simulink model "PID_AccuratePlant"  (R2021a)
settings: Solver=ode45  StartTime=0.0  StopTime=22  RelTol=1e-3
undefined symbols (not defined in the file): drv, gbox, kd_best, ki_best, kp_best, mld, mot, rads2rpm, sens, simp_model
libraries: spsStairGeneratorLib x1
settings Model: Creator=gioel  LastModifiedBy=gioel
settings SolverCC: AlgebraicLoopSolver=TrustRegion
settings DebuggingCC: SFMachineParentedDataDiag=warning

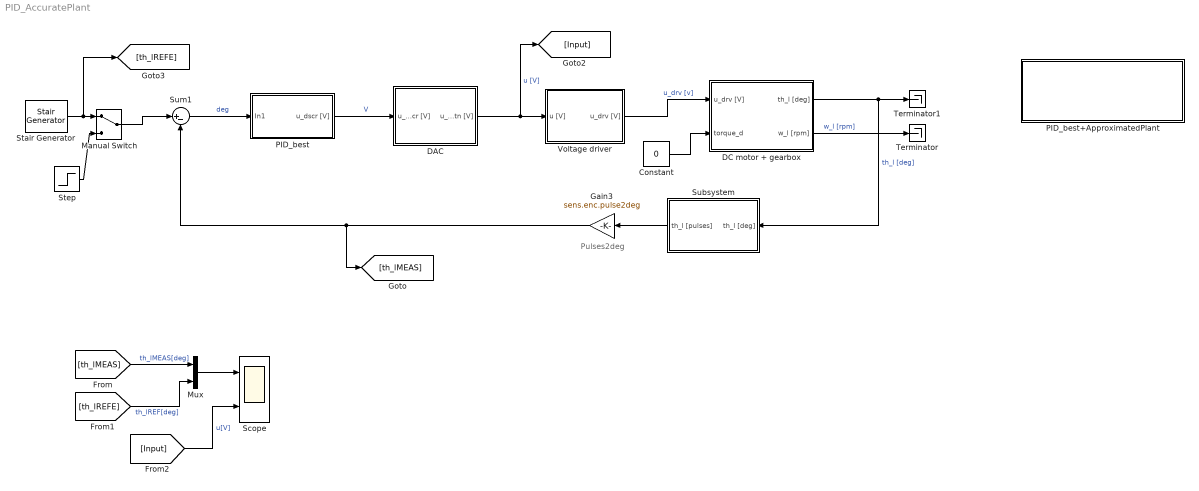
== system PID_AccuratePlant ==
  note: Pulses2deg
  Constant : Constant  Value=0
  DAC : Subsystem
  DC motor + gearbox : Subsystem
  Gain3 : Gain  Gain=sens.enc.pulse2deg
  Manual Switch : ManualSwitch
  Mux : Mux  Inputs=2
  PID_best : Subsystem
  PID_best+ApproximatedPlant : Subsystem
  Scope : Scope  NumInputPorts=2
  Stair Generator : spsStairGeneratorLib/Stair Generator  t=[0,2, 4, 6,8,10,12,14,16,18,20]  e=[10,0,30,0,50,0,90,0,180,0,360]  Ts=0
  Step : Step  Time=0  After=10  SampleTime=0
  Subsystem : Subsystem
  Sum1 : Sum  Inputs=|+-
  Terminator : Terminator
  Terminator1 : Terminator
  Voltage driver : Subsystem
  wires:
  Voltage driver/1(u_drv [V]) -> DC motor + gearbox/1(u_drv [V])  "u_drv [v]"
  DC motor + gearbox/1(th_l [deg]) -> Terminator1/1, Subsystem/1(th_l [deg])  "th_l [deg]"
  DC motor + gearbox/2(w_l [rpm]) -> Terminator/1  "w_l [rpm]"
  DAC/1(u_cntn [V]) -> [Input], Voltage driver/1(u [V])  "u [V]"
  Subsystem/1(th_l [pulses]) -> Gain3/1
  Stair Generator/1 -> [th_lREFE], Manual Switch/1
  Sum1/1 -> PID_best/1(In1)  "deg"
  Gain3/1 -> Sum1/2, [th_lMEAS]
  [th_lMEAS] -> Mux/1  "th_lMEAS[deg]"
  [th_lREFE] -> Mux/2  "th_lREF[deg]"
  [Input] -> Scope/2  "u[V]"
  Mux/1 -> Scope/1
  Step/1 -> Manual Switch/2
  Manual Switch/1 -> Sum1/1
  PID_best/1(u_dscr [V]) -> DAC/1(u_dscr [V])  "V"
  Constant/1 -> DC motor + gearbox/2(torque_d)

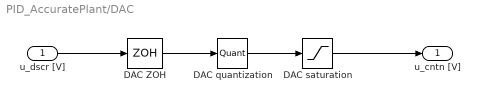
== system PID_AccuratePlant/DAC ==
  u_dscr [V] : Inport
  DAC ZOH : ZeroOrderHold  SampleTime=sens.enc.T_s
  DAC quantization : Quantizer  QuantizationInterval=daq.dac.q
  DAC saturation : Saturate  UpperLimit=10  LowerLimit=-10
  u_cntn [V] : Outport
  wires:
  DAC quantization/1 -> DAC saturation/1
  DAC ZOH/1 -> DAC quantization/1
  DAC saturation/1 -> u_cntn [V]/1
  u_dscr [V]/1 -> DAC ZOH/1

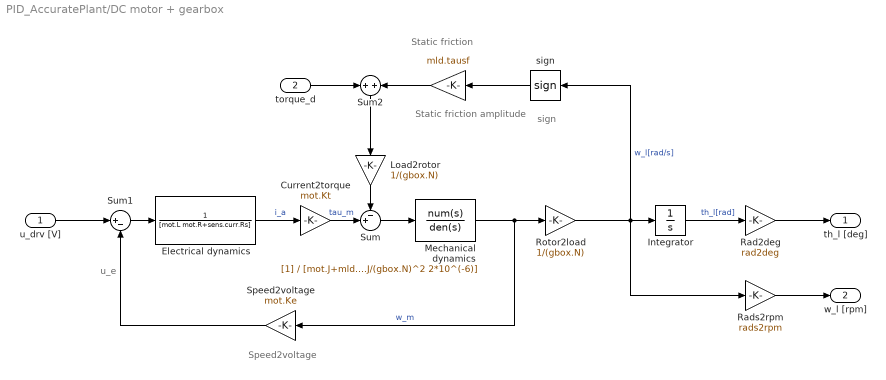
== system PID_AccuratePlant/DC motor + gearbox ==
  note: u_e
  note: Speed2voltage
  note: Static friction
  note: sign
  note: Static friction
      |  amplitude
  u_drv [V] : Inport
  torque_d : Inport  Port=2
  " " : Gain  Gain=mld.tausf
  Current2torque : Gain  Gain=mot.Kt
  Electrical dynamics : TransferFcn  Denominator=[mot.L mot.R+sens.curr.Rs]
  Integrator : Integrator
  Load2rotor : Gain  Gain=1/(gbox.N)
  Mechanical dynamics : TransferFcn  Denominator=[mot.J+mld.J/(gbox.N)^2 2*10^(-6)]
  Rad2deg : Gain  Gain=rad2deg
  Rads2rpm : Gain  Gain=rads2rpm
  Rotor2load : Gain  Gain=1/(gbox.N)
  Speed2voltage : Gain  Gain=mot.Ke
  Sum : Sum  Inputs=-+|
  Sum1 : Sum  Inputs=|+-
  Sum2 : Sum  Inputs=+|+
  sign : Signum  ZeroCross=off
  th_l [deg] : Outport
  w_l [rpm] : Outport  Port=2
  wires:
  u_drv [V]/1 -> Sum1/1
  Rads2rpm/1 -> w_l [rpm]/1
  Electrical dynamics/1 -> Current2torque/1  "i_a"
  Current2torque/1 -> Sum/2  "tau_m"
  Rad2deg/1 -> th_l [deg]/1
  sign/1 -> " "/1
  Sum1/1 -> Electrical dynamics/1
  Integrator/1 -> Rad2deg/1  "th_l[rad]"
  Sum/1 -> Mechanical dynamics/1
  Load2rotor/1 -> Sum/1
  Speed2voltage/1 -> Sum1/2
  Rotor2load/1 -> Rads2rpm/1, sign/1, Integrator/1  "w_l[rad/s]"
  Mechanical dynamics/1 -> Speed2voltage/1, Rotor2load/1  "w_m"
  " "/1 -> Sum2/2
  Sum2/1 -> Load2rotor/1
  torque_d/1 -> Sum2/1

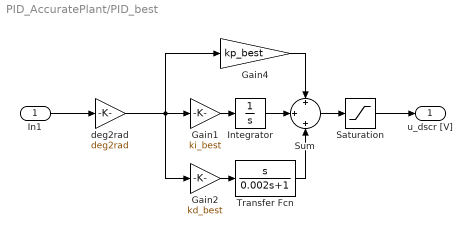
== system PID_AccuratePlant/PID_best ==
  In1 : Inport
  Gain1 : Gain  Gain=ki_best
  Gain2 : Gain  Gain=kd_best
  Gain4 : Gain  Gain=kp_best
  Integrator : Integrator
  Saturation : Saturate  UpperLimit=10  LowerLimit=-10
  Sum : Sum  Inputs=+|+|+
  Transfer Fcn : TransferFcn  Numerator=[1 0]  Denominator=[0.002 1]
  deg2rad : Gain  Gain=deg2rad
  u_dscr [V] : Outport
  wires:
  Transfer Fcn/1 -> Sum/3
  deg2rad/1 -> Gain1/1, Gain4/1, Gain2/1
  In1/1 -> deg2rad/1
  Gain2/1 -> Transfer Fcn/1
  Sum/1 -> Saturation/1
  Saturation/1 -> u_dscr [V]/1
  Integrator/1 -> Sum/2
  Gain1/1 -> Integrator/1
  Gain4/1 -> Sum/1

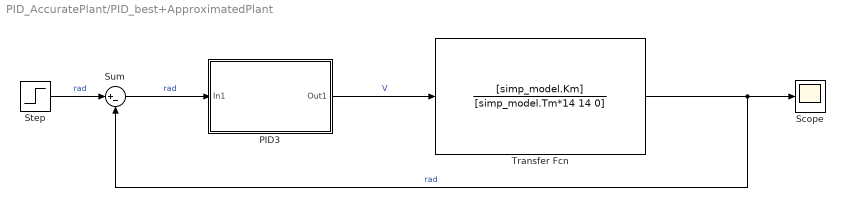
== system PID_AccuratePlant/PID_best+ApproximatedPlant ==
  PID3 : Subsystem
  Scope : Scope
  Step : Step  Time=0  SampleTime=0
  Sum : Sum  Inputs=|+-
  Transfer Fcn : TransferFcn  Numerator=[simp_model.Km]  Denominator=[simp_model.Tm*14 14 0]
  wires:
  PID3/1(Out1) -> Transfer Fcn/1  "V"
  Sum/1 -> PID3/1(In1)  "rad"
  Step/1 -> Sum/1  "rad"
  Transfer Fcn/1 -> Scope/1, Sum/2  "rad"

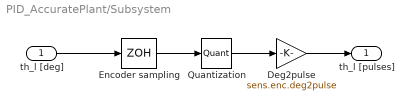
== system PID_AccuratePlant/Subsystem ==
  th_l [deg] : Inport
  Deg2pulse : Gain  Gain=sens.enc.deg2pulse
  Encoder sampling : ZeroOrderHold  SampleTime=0.001
  Quantization : Quantizer  QuantizationInterval=sens.enc.q
  th_l [pulses] : Outport
  wires:
  Encoder sampling/1 -> Quantization/1
  Quantization/1 -> Deg2pulse/1
  th_l [deg]/1 -> Encoder sampling/1
  Deg2pulse/1 -> th_l [pulses]/1

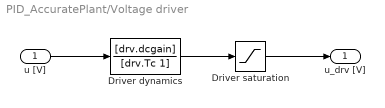
== system PID_AccuratePlant/Voltage driver ==
  u [V] : Inport
  Driver dynamics : TransferFcn  Numerator=[drv.dcgain]  Denominator=[drv.Tc 1]
  Driver saturation : Saturate  UpperLimit=12  LowerLimit=-12
  u_drv [V] : Outport
  wires:
  Driver saturation/1 -> u_drv [V]/1
  Driver dynamics/1 -> Driver saturation/1
  u [V]/1 -> Driver dynamics/1

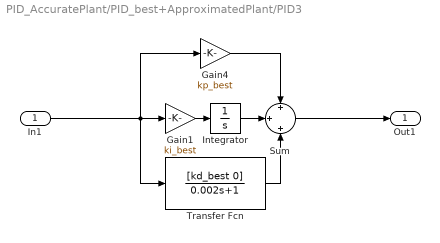
== system PID_AccuratePlant/PID_best+ApproximatedPlant/PID3 ==
  In1 : Inport
  Gain1 : Gain  Gain=ki_best
  Gain4 : Gain  Gain=kp_best
  Integrator : Integrator
  Sum : Sum  Inputs=+|+|+
  Transfer Fcn : TransferFcn  Numerator=[kd_best 0]  Denominator=[0.002 1]
  Out1 : Outport
  wires:
  Gain4/1 -> Sum/1
  Transfer Fcn/1 -> Sum/3
  In1/1 -> Gain1/1, Gain4/1, Transfer Fcn/1
  Sum/1 -> Out1/1
  Integrator/1 -> Sum/2
  Gain1/1 -> Integrator/1
